simulink model "zad2_repr_graf_niel_dyn_mod_dyskretny"  (R2014b)
settings: Solver=ode45  StartTime=0.0  StopTime=10.0  RelTol=1e-3
values from neighbouring files (symbols this model uses):
  a1 = 0.39    [dane_poczatkowe.mat]
  a2 = 0.45    [dane_poczatkowe.mat]
  a3 = -2.91    [dane_poczatkowe.mat]
  a4 = 0.25    [dane_poczatkowe.mat]
  K = 3.5    [dane_poczatkowe.mat]
  T1 = 5    [dane_poczatkowe.mat]
  T2 = 9    [dane_poczatkowe.mat]
  Tp = 0.1    [dane_poczatkowe.mat]
  x1 = 0    [dane_poczatkowe.mat]
  x2 = 0    [dane_poczatkowe.mat]
settings Model: Creator=Konrad  LastModifiedBy=Konrad

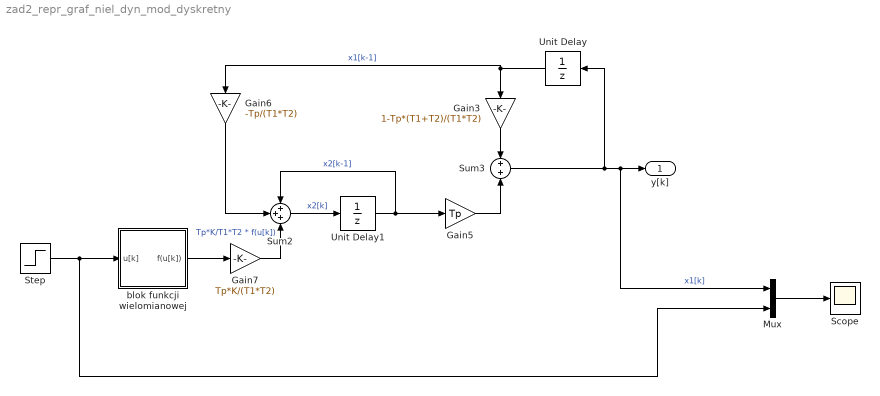
== system zad2_repr_graf_niel_dyn_mod_dyskretny ==
  Gain3 : Gain  Gain=1-Tp*(T1+T2)/(T1*T2)
  Gain5 : Gain  Gain=Tp
  Gain6 : Gain  Gain=-Tp/(T1*T2)
  Gain7 : Gain  Gain=Tp*K/(T1*T2)
  Mux : Mux  Inputs=2
  Scope : Scope
  Step : Step  SampleTime=0
  Sum2 : Sum  Inputs=+++
  Sum3 : Sum  Inputs=+|+
  Unit Delay : UnitDelay  InitialCondition=x1  SampleTime=Tp
  Unit Delay1 : UnitDelay  InitialCondition=x2  SampleTime=Tp
  blok funkcji wielomianowej : Subsystem
  y[k] : Outport
  wires:
  Sum3/1 -> Unit Delay/1, Mux/1, y[k]/1  "x1[k]"
  Unit Delay/1 -> Gain6/1, Gain3/1  "x1[k-1]"
  Gain3/1 -> Sum3/1
  Unit Delay1/1 -> Gain5/1, Sum2/1  "x2[k-1]"
  Gain5/1 -> Sum3/2
  Sum2/1 -> Unit Delay1/1  "x2[k]"
  Gain6/1 -> Sum2/2
  Step/1 -> Mux/2, blok funkcji wielomianowej/1(u[k])
  blok funkcji wielomianowej/1(f(u[k])) -> Gain7/1
  Gain7/1 -> Sum2/3  "Tp*K/T1*T2 * f(u[k])"
  Mux/1 -> Scope/1

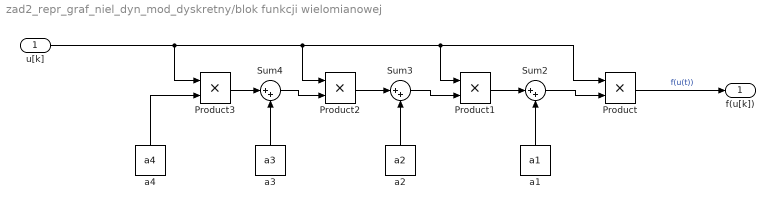
== system zad2_repr_graf_niel_dyn_mod_dyskretny/blok funkcji wielomianowej ==
  u[k] : Inport
  Product{,1..3} (4 alike) : Product
  Sum2 : Sum  Inputs=|++
  Sum3 : Sum  Inputs=|++
  Sum4 : Sum  Inputs=|++
  a1 : Constant  Value=a1
  a2 : Constant  Value=a2
  a3 : Constant  Value=a3
  a4 : Constant  Value=a4
  f(u[k]) : Outport
  wires:
  u[k]/1 -> Product/1, Product1/1, Product2/1, Product3/1
  Product1/1 -> Sum2/1
  Product2/1 -> Sum3/1
  Sum2/1 -> Product/2
  Product/1 -> f(u[k])/1  "f(u(t))"
  Product3/1 -> Sum4/1
  a1/1 -> Sum2/2
  a2/1 -> Sum3/2
  Sum3/1 -> Product1/2
  a3/1 -> Sum4/2
  Sum4/1 -> Product2/2
  a4/1 -> Product3/2
